simulink subsystem "ControladorBorroso_parte2"  (R2019b)
settings: Solver=VariableStepAuto  StartTime=0.0  StopTime=10.0  RelTol=1e-3
libraries: fuzblock x1, simulink x1
settings Model: Creator=laura  LastModifiedBy=laura

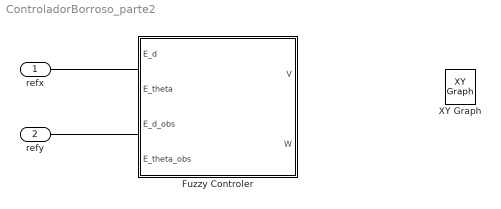
== system ControladorBorroso_parte2 ==
  "refx " : Inport
  refy : Inport  Port=2
  Fuzzy Controler : Subsystem
  XY Graph : simulink/Sinks/XY Graph  xmin=-5  xmax=5  ymin=-5  ymax=5  st=-1
  wires:
  "refx "/1 -> ?
  refy/1 -> ?
  ? -> XY Graph/1
  ? -> XY Graph/2

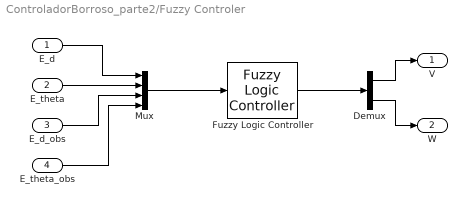
== system ControladorBorroso_parte2/Fuzzy Controler ==
  E_d : Inport
  E_theta : Inport  Port=2
  E_d_obs : Inport  Port=3
  E_theta_obs : Inport  Port=4
  Demux : Demux  Outputs=2
  Fuzzy Logic Controller : fuzblock/Fuzzy Logic  Controller  FIS='ControlBorrosoObs.fis'  OutputSampleNumber=101  DataType=double  FuzzifiedInputs=off  RuleFiringStrengths=off  RuleOutputs=off  AggregatedOutputs=off  SimulateUsing=Interpreted execution  OutOfRangeInputValueMessage=warning  NoRuleFiredMessage=warning  EmptyOutputFuzzySetMessage=warning
  Mux : Mux
  V : Outport  VectorParamsAs1DForOutWhenUnconnected=off
  W : Outport  Port=2  VectorParamsAs1DForOutWhenUnconnected=off
  wires:
  Mux/1 -> Fuzzy Logic Controller/1
  E_theta/1 -> Mux/2
  Fuzzy Logic Controller/1 -> Demux/1
  Demux/1 -> V/1
  E_theta_obs/1 -> Mux/4
  E_d/1 -> Mux/1
  Demux/2 -> W/1
  E_d_obs/1 -> Mux/3
